simulink model "RobotLib"  (R2018b)
settings: Solver=ode5  StartTime=0.0  StopTime=10  FixedStep=0.0001  RelTol=1e-3
PreLoadFcn:
  | load('Arm6SimscapeData.mat');
model workspace: external: MAT-File E:\SixRobotArm\Simscape_Simulation\StepFile\Arm6Assembly_DataFile.mat (data not in the file)
values from neighbouring files (symbols this model uses):
  smiData =     [Arm6SimscapeData.mat]
undefined symbols (not defined in the file or in its folder): X, Y, Z
libraries: sm_lib x216, nesl_utility x186, fl_lib x114
(part 1 of 6)
settings Model: Creator=Administrator  LastModifiedBy=Jeason
settings SolverCC: AutoInsertRateTranBlk=on
settings DataIOCC: ReturnWorkspaceOutputs=on
settings ExplorerConfigSet: InternalSimMechanicsExplorerSettings="<ExplorerConfiguration><canonicalview>planar_xy</canonicalview><AnimationSetting><BasePlaybackSpeed>1.0</BasePlaybackSpeed><PlaybackSpeedFactor>1.0</PlaybackSpeedFactor></AnimationSetting><TilePanel><TileInfo><Tiles Columns=\"1\" Count=\"1\" Rows=\"1\"><Column Weight=\"1\"/><Row Weight=\"1\"/><Tile Height=\"1\" Width=\"1\" X=\"0\" Y=\"0\"/></Tiles></TileInfo><SceneInfo><SceneViewer><BGColor><R>0.60000002384185791</R><G>0.60000002384185791</G><B>0.60000002384185791</B></BGColor><Camera><DoPerspective>off</DoPerspective><Position><X>0.529425685588477024</X><Y>0.96968881474758839</Y><Z>0.531520526083879341</Z></Position><Center><X>-0.0479245836011489429</X><Y>0.392338545557962604</Y><Z>-0.0458297431057466537</Z></Center><Up><X>-0.408248290463863073</X><Y>0.816496580927726145</Y><Z>-0.408248290463863073</Z></Up><ViewLimDist>1</ViewLimDist><YLim>0.78131541566616991</YLim><XLim>0.557104420151891211</XLim></Camera></SceneViewer></SceneInfo></TilePanel><MechEditorPanel><Cameras/><GfxPanelCameraMap/><VideoCreator><PlaybackSpeedRatio>1.0</PlaybackSpeedRatio><FrameRate>30</FrameRate><VideoFormat>MPEG-4</VideoFormat><FrameSize>[400 400]</FrameSize></VideoCreator></MechEditorPanel></ExplorerConfiguration>"

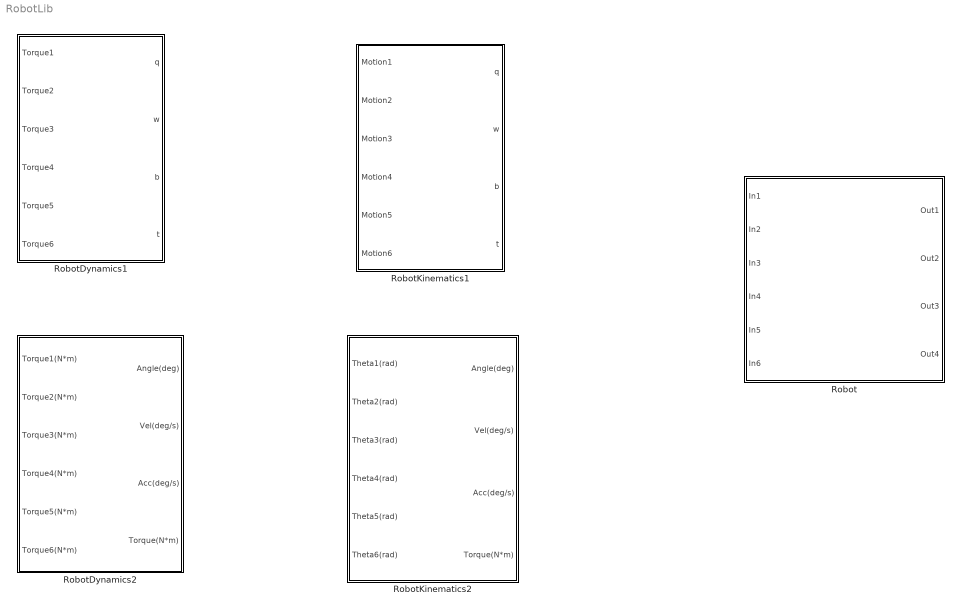
== system RobotLib ==
  Robot : Subsystem  mask(模式选择){VChoice=Kinematics}
      mask prompts: VChoice "Select a variant choice"
      mask help: 选择运动学Simscape模型或者动力学Simscape模型
      mask init:
      | %     simulationStatus =  get_param(bdroot,'SimulationStatus');
      | % 
      | % % The active variant can only be modified at edit-time or very early during
      | % % the simulink compile stage. 
      | %     choice = get_param(gcb,'VChoice');
      | %     vssBlk = [gcb, '/VariantSubsystem'];
      | %     oldVariant = get_param(gcb,'OverrideUsingVariant');
      | % 
      | %     if strcmp(choice,'Kinematics')
      | %         port_label('input', 1, 'Theta1(rad)');
      | %         port_label('input', 2, 'Theta2(rad)');
      | %         port_label('input', 3, 'Theta3(rad)');
      | %         port_label('input', 4, 'Theta4(rad)');
      | %         port_label('input', 5, 'Theta5(rad)');
      | %         port_label('input', 6, 'Theta6(rad)');
      | %         set_param(vssBlk, 'OverrideUsingVariant', 'Variant1');
      | %     else
      | %         port_label('input', 1, 'Torque1(N*m)');
      | %         port_label('input', 2, 'Torque2(N*m)');
      | %         port_label('input', 3, 'Torque3(N*m)');
      | %         port_label('input', 4, 'Torque4(N*m)');
      | %         port_label('input', 5, 'Torque5(N*m)');
      | %         port_label('input', 6, 'Torque6(N*m)');
      | %         set_param(vssBlk, 'OverrideUsingVariant', 'Variant2');
      | %     end
      mask TypeOptions VChoice: Kinematics | Dynamics
      mask Display:
      | image('E:\SixRobotArm\Robot.png') ;
      | simulationStatus =  get_param(bdroot,'SimulationStatus');
      | % The active variant can only be modified at edit-time or very early during
      | % the simulink compile stage.
      |     choice = get_param(gcb,'VChoice');
      |     vssBlk = [gcb, '/VariantSubsystem'];
      |     oldVariant = get_param(gcb,'OverrideUsingVariant');
      | if strcmp(choice,'Kinematics')
      |     port_label('input', 1, 'Theta1(rad)');
      |     port_label('input', 2, 'Theta2(rad)');
      |     port_label('input', 3, 'Theta3(rad)');
      |     port_label('input', 4, 'Theta4(rad)');
      |     port_label('input', 5, 'Theta5(rad)');
      |     port_label('input', 6, 'Theta6(rad)');
      |     set_param(vssBlk, 'OverrideUsingVariant', 'Variant1');
      | else
      |     port_label('input', 1, 'Torque1(N*m)');
      |     port_label('input', 2, 'Torque2(N*m)');
      |     port_label('input', 3, 'Torque3(N*m)');
      |     port_label('input', 4, 'Torque4(N*m)');
      |     port_label('input', 5, 'Torque5(N*m)');
      |     port_label('input', 6, 'Torque6(N*m)');
      |     set_param(vssBlk, 'OverrideUsingVariant', 'Variant2');
      | end
      | 
      | port_label('output', 1, 'Angle(deg)');
      | port_label('output', 2, 'Vel(deg/s)');
      | port_label('output', 3, 'Acc(deg/s^2)');
      | port_label('output', 4, 'Torque(N*m)');
  RobotDynamics1 : Subsystem
  RobotDynamics2 : Subsystem
  RobotKinematics1 : Subsystem
  RobotKinematics2 : Subsystem

== system RobotLib/Robot ==
  In1 : Inport
  In2 : Inport  Port=2
  In3 : Inport  Port=3
  In4 : Inport  Port=4
  In5 : Inport  Port=5
  In6 : Inport  Port=6
  VariantSubsystem : Subsystem  VariantControlMode=Label  Variant=on  LabelModeActiveChoice=Variant1
  Out1 : Outport
  Out2 : Outport  Port=2
  Out3 : Outport  Port=3
  Out4 : Outport  Port=4
  wires:
  VariantSubsystem/1(Out1) -> Out1/1
  In5/1 -> VariantSubsystem/5(In5)
  In1/1 -> VariantSubsystem/1(In1)
  In4/1 -> VariantSubsystem/4(In4)
  In6/1 -> VariantSubsystem/6(In6)
  In2/1 -> VariantSubsystem/2(In2)
  In3/1 -> VariantSubsystem/3(In3)
  VariantSubsystem/2(Out2) -> Out2/1
  VariantSubsystem/3(Out3) -> Out3/1
  VariantSubsystem/4(Out4) -> Out4/1

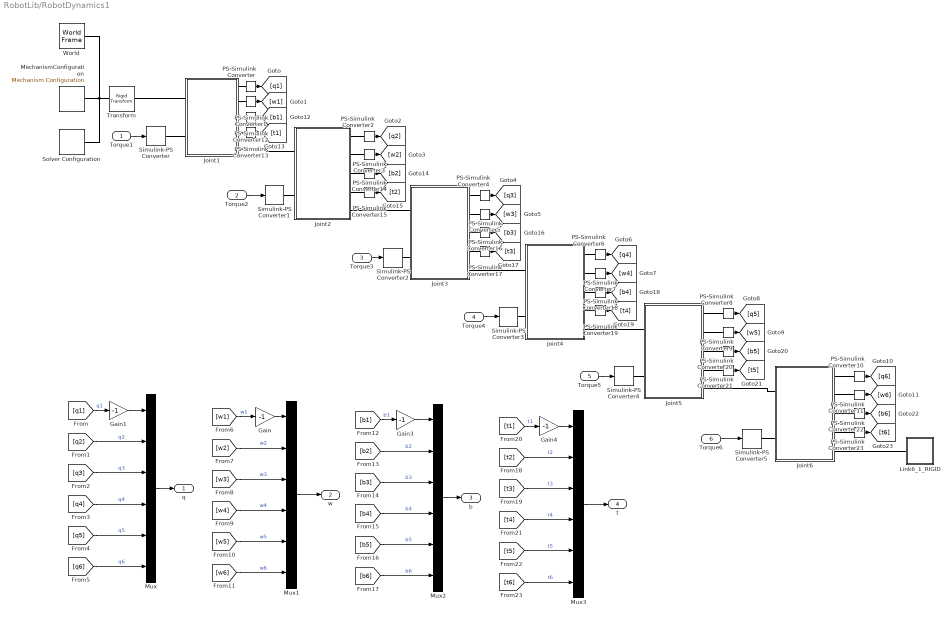
== system RobotLib/RobotDynamics1 ==
  Torque1 : Inport
  Torque2 : Inport  Port=2
  Torque3 : Inport  Port=3
  Torque4 : Inport  Port=4
  Torque5 : Inport  Port=5
  Torque6 : Inport  Port=6
  Gain{,1,3..4} (4 alike) : Gain  Gain=-1
  Joint1 : Subsystem
  Joint2 : Subsystem
  Joint3 : Subsystem
  Joint4 : Subsystem
  Joint5 : Subsystem
  Joint6 : Subsystem
  Link6_1_RIGID : Subsystem
  MechanismConfiguration : sm_lib/Utilities/Mechanism Configuration  UniformGravity=Constant  GravityVector=[0 -9.80665 0]  GravityUnits=m/s^2  LinearizationDelta=0.001
  Mux{,1..3} (4 alike) : Mux  Inputs=6
  PS-Simulink Converter{,2,4,6,8,10} (6 alike) : nesl_utility/PS-Simulink Converter  PhysicalDomain=network_engine_domain  SubClassName=ps_output  LeftPortType=input  RightPortType=output  PseudoPeriodic=off  Frequencies=[]  Unit=deg  AffineConversion=off
  PS-Simulink Converter{1,3,5,7,9,11} (6 alike) : nesl_utility/PS-Simulink Converter  PhysicalDomain=network_engine_domain  SubClassName=ps_output  LeftPortType=input  RightPortType=output  PseudoPeriodic=off  Frequencies=[]  Unit=deg/s  AffineConversion=off
  PS-Simulink Converter{12,14,16,18,20,22} (6 alike) : nesl_utility/PS-Simulink Converter  PhysicalDomain=network_engine_domain  SubClassName=ps_output  LeftPortType=input  RightPortType=output  PseudoPeriodic=off  Frequencies=[]  Unit=deg/s^2  AffineConversion=off
  PS-Simulink Converter{13,15,17,19,21,23} (6 alike) : nesl_utility/PS-Simulink Converter  PhysicalDomain=network_engine_domain  SubClassName=ps_output  LeftPortType=input  RightPortType=output  PseudoPeriodic=off  Frequencies=[]  Unit=N*m  AffineConversion=off
  Simulink-PS Converter{,1..5} (6 alike) : nesl_utility/Simulink-PS Converter  PhysicalDomain=network_engine_domain  SubClassName=ps_input  LeftPortType=input  RightPortType=output  PseudoPeriodic=off  Frequencies=[]  NoiseDistribution=none  NoiseParameters=[]  Unit=N*m  AffineConversion=off  FilteringAndDerivatives=provide  SimscapeFilterOrder=2  InputFilterTimeConstant=0.001  UdotUserProvided=0
  Solver Configuration : nesl_utility/Solver Configuration  PhysicalDomain=network_engine_domain  SubClassName=solver  LeftPortType=input  RightPortType=generic  Tones=[]  Harmonics=[]  SimulateNoise=off  Profile=off  UseLocalSampling=off  EnableSwitchedLinearOptims=on  FrequencyDomain=off  UseCCode=off  RelTol=0.001  AbsTol=1e-06  MinStep=1e-09  ToWorkspace=off  RevertToSquareIcSolve=off  NumHomotopyIterations=100  PhasorMode=off  PhasorModeNumHarmonics=1  DoDC=off  ResidualTolerance=1e-09  UseLocalSolver=off  LocalSolverChoice=NE_BACKWARD_EULER_ADVANCER  LocalSolverSampleTime=0.001  DoFixedCost=off  MaxNonlinIter=3  MaxModeIter=2  LinearAlgebra=auto  EquationFormulation=NE_TIME_EF  DelaysMemoryBudget=1024  AutomaticFiltering=on  FilteringTimeConstant=0.001  PartitionStorageMethod=AS_NEEDED  PartitionMemoryBudget=1024
  Transform : sm_lib/Frames and Transforms/Rigid Transform  TranslationMethod=Cartesian  TranslationStandardOffset=0  TranslationLengthUnit=mm  TranslationStandardAxis=+Z  TranslationCartesianOffset=smiData.RigidTransform(14).translation  TranslationROffset=0  TranslationROffsetUnits=m  TranslationZOffset=0  TranslationZOffsetUnits=m  TranslationThetaOffset=0  TranslationThetaOffsetUnits=deg  RotationMethod=ArbitraryAxis  RotationAngleUnits=rad  RotationStandardAxis=+Z  RotationAngle=smiData.RigidTransform(14).angle  RotationArbitraryAxis=smiData.RigidTransform(14).axis  FollAlignAxisA=+X  BaseAlignAxisA=+Y  FollAlignAxisB=+Y  BaseAlignAxisB=+Z  RotationSequenceAxes=FollowerAxes  RotationSequence=XYX  RotationSequenceAngles=[0 0 0]  RotationSequenceAnglesUnits=deg  RotationMatrix=[1 0 0; 0 1 0; 0 0 1]
  World : sm_lib/Frames and Transforms/World Frame
  q : Outport  VectorParamsAs1DForOutWhenUnconnected=on
  w : Outport  Port=2  VectorParamsAs1DForOutWhenUnconnected=on
  b : Outport  Port=3  VectorParamsAs1DForOutWhenUnconnected=on
  t : Outport  Port=4  VectorParamsAs1DForOutWhenUnconnected=on
  wires:
  [q5] -> Mux/5  "q5"
  Mux/1 -> q/1
  PS-Simulink Converter6/1 -> [q4]
  [w4] -> Mux1/4  "w4"
  PS-Simulink Converter/1 -> [q1]
  [q6] -> Mux/6  "q6"
  [w1] -> Gain/1  "w1"
  [w5] -> Mux1/5  "w5"
  PS-Simulink Converter4/1 -> [q3]
  PS-Simulink Converter5/1 -> [w3]
  PS-Simulink Converter9/1 -> [w5]
  [w2] -> Mux1/2  "w2"
  PS-Simulink Converter1/1 -> [w1]
  [q2] -> Mux/2  "q2"
  PS-Simulink Converter10/1 -> [q6]
  [w6] -> Mux1/6  "w6"
  PS-Simulink Converter7/1 -> [w4]
  [q4] -> Mux/4  "q4"
  PS-Simulink Converter11/1 -> [w6]
  PS-Simulink Converter8/1 -> [q5]
  Mux1/1 -> w/1
  PS-Simulink Converter2/1 -> [q2]
  [q3] -> Mux/3  "q3"
  [q1] -> Gain1/1  "q1"
  [w3] -> Mux1/3  "w3"
  PS-Simulink Converter3/1 -> [w2]
  Torque2/1 -> Simulink-PS Converter1/1
  Torque3/1 -> Simulink-PS Converter2/1
  Torque4/1 -> Simulink-PS Converter3/1
  Torque5/1 -> Simulink-PS Converter4/1
  Torque6/1 -> Simulink-PS Converter5/1
  Gain/1 -> Mux1/1
  Gain1/1 -> Mux/1
  PS-Simulink Converter12/1 -> [b1]
  PS-Simulink Converter13/1 -> [t1]
  PS-Simulink Converter15/1 -> [t2]
  PS-Simulink Converter14/1 -> [b2]
  PS-Simulink Converter16/1 -> [b3]
  PS-Simulink Converter17/1 -> [t3]
  PS-Simulink Converter19/1 -> [t4]
  PS-Simulink Converter18/1 -> [b4]
  PS-Simulink Converter20/1 -> [b5]
  PS-Simulink Converter21/1 -> [t5]
  PS-Simulink Converter23/1 -> [t6]
  PS-Simulink Converter22/1 -> [b6]
  Gain3/1 -> Mux2/1
  [b1] -> Gain3/1  "b1"
  Mux3/1 -> t/1
  [t1] -> Gain4/1  "t1"
  Mux2/1 -> b/1
  [b2] -> Mux2/2  "b2"
  [b3] -> Mux2/3  "b3"
  [b4] -> Mux2/4  "b4"
  [b5] -> Mux2/5  "b5"
  [b6] -> Mux2/6  "b6"
  [t2] -> Mux3/2  "t2"
  [t3] -> Mux3/3  "t3"
  [t4] -> Mux3/4  "t4"
  [t5] -> Mux3/5  "t5"
  [t6] -> Mux3/6  "t6"
  Torque1/1 -> Simulink-PS Converter/1
  Gain4/1 -> Mux3/1
  connections:
  Joint6/RConn1 -- PS-Simulink Converter10/LConn1
  PS-Simulink Converter11/LConn1 -- Joint6/RConn2
  Joint4/RConn2 -- PS-Simulink Converter7/LConn1
  Joint4/RConn1 -- PS-Simulink Converter6/LConn1
  PS-Simulink Converter9/LConn1 -- Joint5/RConn2
  PS-Simulink Converter5/LConn1 -- Joint3/RConn2
  Transform/LConn1 -- MechanismConfiguration/RConn1 -- Solver Configuration/RConn1 -- World/RConn1
  Joint3/RConn5 -- Joint4/LConn1
  Joint1/RConn2 -- PS-Simulink Converter1/LConn1
  PS-Simulink Converter3/LConn1 -- Joint2/RConn2
  Joint1/LConn1 -- Transform/RConn1
  PS-Simulink Converter8/LConn1 -- Joint5/RConn1
  Simulink-PS Converter3/RConn1 -- Joint4/LConn2
  PS-Simulink Converter4/LConn1 -- Joint3/RConn1
  Joint1/RConn1 -- PS-Simulink Converter/LConn1
  Joint6/LConn1 -- Joint5/RConn5
  Joint3/LConn1 -- Joint2/RConn5
  Joint5/LConn1 -- Joint4/RConn5
  Link6_1_RIGID/LConn1 -- Joint6/RConn5
  Simulink-PS Converter5/RConn1 -- Joint6/LConn2
  Simulink-PS Converter1/RConn1 -- Joint2/LConn2
  PS-Simulink Converter2/LConn1 -- Joint2/RConn1
  Joint5/LConn2 -- Simulink-PS Converter4/RConn1
  Joint2/LConn1 -- Joint1/RConn5
  Simulink-PS Converter2/RConn1 -- Joint3/LConn2
  PS-Simulink Converter12/LConn1 -- Joint1/RConn3
  PS-Simulink Converter13/LConn1 -- Joint1/RConn4
  PS-Simulink Converter15/LConn1 -- Joint2/RConn4
  PS-Simulink Converter14/LConn1 -- Joint2/RConn3
  PS-Simulink Converter16/LConn1 -- Joint3/RConn3
  Joint3/RConn4 -- PS-Simulink Converter17/LConn1
  PS-Simulink Converter18/LConn1 -- Joint4/RConn3
  PS-Simulink Converter19/LConn1 -- Joint4/RConn4
  PS-Simulink Converter20/LConn1 -- Joint5/RConn3
  PS-Simulink Converter21/LConn1 -- Joint5/RConn4
  PS-Simulink Converter23/LConn1 -- Joint6/RConn4
  Joint6/RConn3 -- PS-Simulink Converter22/LConn1
  Joint1/LConn2 -- Simulink-PS Converter/RConn1

== system RobotLib/RobotDynamics2 ==
  Torque1(N*m) : Inport
  Torque2(N*m) : Inport  Port=2
  Torque3(N*m) : Inport  Port=3
  Torque4(N*m) : Inport  Port=4
  Torque5(N*m) : Inport  Port=5
  Torque6(N*m) : Inport  Port=6
  RobotDynamics1 : Subsystem
  Angle(deg) : Outport
  Vel(deg/s) : Outport  Port=2
  Acc(deg/s) : Outport  Port=3
  Torque(N*m) : Outport  Port=4
  wires:
  Torque5(N*m)/1 -> RobotDynamics1/5(Torque5)
  Torque2(N*m)/1 -> RobotDynamics1/2(Torque2)
  Torque3(N*m)/1 -> RobotDynamics1/3(Torque3)
  Torque6(N*m)/1 -> RobotDynamics1/6(Torque6)
  RobotDynamics1/1(q) -> Angle(deg)/1
  Torque1(N*m)/1 -> RobotDynamics1/1(Torque1)
  Torque4(N*m)/1 -> RobotDynamics1/4(Torque4)
  RobotDynamics1/2(w) -> Vel(deg/s)/1
  RobotDynamics1/3(b) -> Acc(deg/s)/1
  RobotDynamics1/4(t) -> Torque(N*m)/1

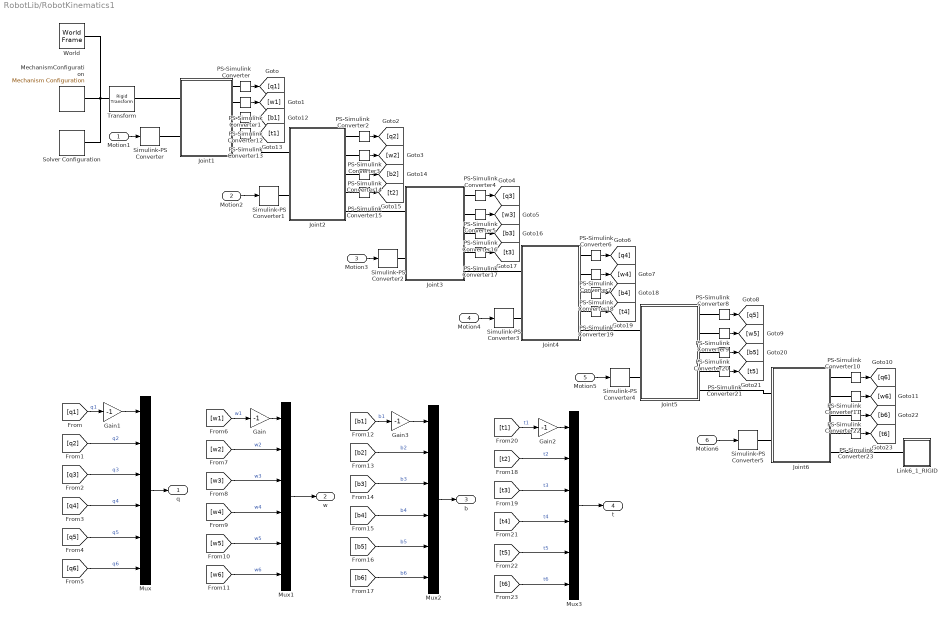
== system RobotLib/RobotKinematics1 ==
  Motion1 : Inport
  Motion2 : Inport  Port=2
  Motion3 : Inport  Port=3
  Motion4 : Inport  Port=4
  Motion5 : Inport  Port=5
  Motion6 : Inport  Port=6
  Gain{,1..3} (4 alike) : Gain  Gain=-1
  Joint1 : Subsystem
  Joint2 : Subsystem
  Joint3 : Subsystem
  Joint4 : Subsystem
  Joint5 : Subsystem
  Joint6 : Subsystem
  Link6_1_RIGID : Subsystem
  MechanismConfiguration : sm_lib/Utilities/Mechanism Configuration  UniformGravity=Constant  GravityVector=[0 -9.80665 0]  GravityUnits=m/s^2  LinearizationDelta=0.001
  Mux{,1..3} (4 alike) : Mux  Inputs=6
  PS-Simulink Converter{,2,4,6,8,10} (6 alike) : nesl_utility/PS-Simulink Converter  PhysicalDomain=network_engine_domain  SubClassName=ps_output  LeftPortType=input  RightPortType=output  PseudoPeriodic=off  Frequencies=[]  Unit=deg  AffineConversion=off
  PS-Simulink Converter{1,3,5,7,9,11} (6 alike) : nesl_utility/PS-Simulink Converter  PhysicalDomain=network_engine_domain  SubClassName=ps_output  LeftPortType=input  RightPortType=output  PseudoPeriodic=off  Frequencies=[]  Unit=deg/s  AffineConversion=off
  PS-Simulink Converter{12,14,16,18,20,22} (6 alike) : nesl_utility/PS-Simulink Converter  PhysicalDomain=network_engine_domain  SubClassName=ps_output  LeftPortType=input  RightPortType=output  PseudoPeriodic=off  Frequencies=[]  Unit=deg/s^2  AffineConversion=off
  PS-Simulink Converter{13,15,17,19,21,23} (6 alike) : nesl_utility/PS-Simulink Converter  PhysicalDomain=network_engine_domain  SubClassName=ps_output  LeftPortType=input  RightPortType=output  PseudoPeriodic=off  Frequencies=[]  Unit=N*m  AffineConversion=off
  Simulink-PS Converter{,1..5} (6 alike) : nesl_utility/Simulink-PS Converter  PhysicalDomain=network_engine_domain  SubClassName=ps_input  LeftPortType=input  RightPortType=output  PseudoPeriodic=off  Frequencies=[]  NoiseDistribution=none  NoiseParameters=[]  Unit=rad  AffineConversion=off  FilteringAndDerivatives=provide  SimscapeFilterOrder=2  InputFilterTimeConstant=0.001  UdotUserProvided=0
  Solver Configuration : nesl_utility/Solver Configuration  PhysicalDomain=network_engine_domain  SubClassName=solver  LeftPortType=input  RightPortType=generic  Tones=[]  Harmonics=[]  SimulateNoise=off  Profile=off  UseLocalSampling=off  EnableSwitchedLinearOptims=on  FrequencyDomain=off  UseCCode=off  RelTol=0.001  AbsTol=1e-06  MinStep=1e-09  ToWorkspace=off  RevertToSquareIcSolve=off  NumHomotopyIterations=100  PhasorMode=off  PhasorModeNumHarmonics=1  DoDC=off  ResidualTolerance=1e-09  UseLocalSolver=off  LocalSolverChoice=NE_BACKWARD_EULER_ADVANCER  LocalSolverSampleTime=0.001  DoFixedCost=off  MaxNonlinIter=3  MaxModeIter=2  LinearAlgebra=auto  EquationFormulation=NE_TIME_EF  DelaysMemoryBudget=1024  AutomaticFiltering=on  FilteringTimeConstant=0.001  PartitionStorageMethod=AS_NEEDED  PartitionMemoryBudget=1024
  Transform : sm_lib/Frames and Transforms/Rigid Transform  TranslationMethod=Cartesian  TranslationStandardOffset=0  TranslationLengthUnit=mm  TranslationStandardAxis=+Z  TranslationCartesianOffset=smiData.RigidTransform(14).translation  TranslationROffset=0  TranslationROffsetUnits=m  TranslationZOffset=0  TranslationZOffsetUnits=m  TranslationThetaOffset=0  TranslationThetaOffsetUnits=deg  RotationMethod=ArbitraryAxis  RotationAngleUnits=rad  RotationStandardAxis=+Z  RotationAngle=smiData.RigidTransform(14).angle  RotationArbitraryAxis=smiData.RigidTransform(14).axis  FollAlignAxisA=+X  BaseAlignAxisA=+Y  FollAlignAxisB=+Y  BaseAlignAxisB=+Z  RotationSequenceAxes=FollowerAxes  RotationSequence=XYX  RotationSequenceAngles=[0 0 0]  RotationSequenceAnglesUnits=deg  RotationMatrix=[1 0 0; 0 1 0; 0 0 1]
  World : sm_lib/Frames and Transforms/World Frame
  q : Outport  VectorParamsAs1DForOutWhenUnconnected=on
  w : Outport  Port=2  VectorParamsAs1DForOutWhenUnconnected=on
  b : Outport  Port=3  VectorParamsAs1DForOutWhenUnconnected=on
  t : Outport  Port=4  VectorParamsAs1DForOutWhenUnconnected=on
  wires:
  [t6] -> Mux3/6  "t6"
  [t5] -> Mux3/5  "t5"
  [t4] -> Mux3/4  "t4"
  [t3] -> Mux3/3  "t3"
  [t2] -> Mux3/2  "t2"
  [b6] -> Mux2/6  "b6"
  [b5] -> Mux2/5  "b5"
  [b4] -> Mux2/4  "b4"
  [b3] -> Mux2/3  "b3"
  [b2] -> Mux2/2  "b2"
  Mux2/1 -> b/1
  [t1] -> Gain2/1  "t1"
  Mux3/1 -> t/1
  [b1] -> Gain3/1  "b1"
  Gain2/1 -> Mux3/1
  Gain3/1 -> Mux2/1
  PS-Simulink Converter22/1 -> [b6]
  PS-Simulink Converter23/1 -> [t6]
  PS-Simulink Converter21/1 -> [t5]
  PS-Simulink Converter20/1 -> [b5]
  PS-Simulink Converter18/1 -> [b4]
  PS-Simulink Converter19/1 -> [t4]
  PS-Simulink Converter17/1 -> [t3]
  PS-Simulink Converter16/1 -> [b3]
  PS-Simulink Converter14/1 -> [b2]
  PS-Simulink Converter15/1 -> [t2]
  PS-Simulink Converter13/1 -> [t1]
  PS-Simulink Converter12/1 -> [b1]
  Gain1/1 -> Mux/1
  Gain/1 -> Mux1/1
  Motion6/1 -> Simulink-PS Converter5/1
  Motion5/1 -> Simulink-PS Converter4/1
  Motion4/1 -> Simulink-PS Converter3/1
  Motion3/1 -> Simulink-PS Converter2/1
  Motion2/1 -> Simulink-PS Converter1/1
  Motion1/1 -> Simulink-PS Converter/1
  PS-Simulink Converter3/1 -> [w2]
  [w3] -> Mux1/3  "w3"
  [q1] -> Gain1/1  "q1"
  [q3] -> Mux/3  "q3"
  PS-Simulink Converter2/1 -> [q2]
  Mux1/1 -> w/1
  PS-Simulink Converter8/1 -> [q5]
  PS-Simulink Converter11/1 -> [w6]
  [q4] -> Mux/4  "q4"
  PS-Simulink Converter7/1 -> [w4]
  [w6] -> Mux1/6  "w6"
  PS-Simulink Converter10/1 -> [q6]
  [q2] -> Mux/2  "q2"
  PS-Simulink Converter1/1 -> [w1]
  [w2] -> Mux1/2  "w2"
  PS-Simulink Converter9/1 -> [w5]
  PS-Simulink Converter5/1 -> [w3]
  PS-Simulink Converter4/1 -> [q3]
  [w5] -> Mux1/5  "w5"
  [w1] -> Gain/1  "w1"
  [q6] -> Mux/6  "q6"
  PS-Simulink Converter/1 -> [q1]
  [w4] -> Mux1/4  "w4"
  PS-Simulink Converter6/1 -> [q4]
  Mux/1 -> q/1
  [q5] -> Mux/5  "q5"
  connections:
  Joint6/RConn3 -- PS-Simulink Converter22/LConn1
  PS-Simulink Converter23/LConn1 -- Joint6/RConn4
  PS-Simulink Converter21/LConn1 -- Joint5/RConn4
  PS-Simulink Converter20/LConn1 -- Joint5/RConn3
  PS-Simulink Converter19/LConn1 -- Joint4/RConn4
  PS-Simulink Converter18/LConn1 -- Joint4/RConn3
  Joint3/RConn4 -- PS-Simulink Converter17/LConn1
  PS-Simulink Converter16/LConn1 -- Joint3/RConn3
  PS-Simulink Converter14/LConn1 -- Joint2/RConn3
  PS-Simulink Converter15/LConn1 -- Joint2/RConn4
  PS-Simulink Converter13/LConn1 -- Joint1/RConn4
  PS-Simulink Converter12/LConn1 -- Joint1/RConn3
  Joint1/LConn2 -- Simulink-PS Converter/RConn1
  Simulink-PS Converter2/RConn1 -- Joint3/LConn2
  Joint2/LConn1 -- Joint1/RConn5
  Joint5/LConn2 -- Simulink-PS Converter4/RConn1
  PS-Simulink Converter2/LConn1 -- Joint2/RConn1
  Simulink-PS Converter1/RConn1 -- Joint2/LConn2
  Simulink-PS Converter5/RConn1 -- Joint6/LConn2
  Link6_1_RIGID/LConn1 -- Joint6/RConn5
  Joint5/LConn1 -- Joint4/RConn5
  Joint3/LConn1 -- Joint2/RConn5
  Joint6/LConn1 -- Joint5/RConn5
  Joint1/RConn1 -- PS-Simulink Converter/LConn1
  PS-Simulink Converter4/LConn1 -- Joint3/RConn1
  Simulink-PS Converter3/RConn1 -- Joint4/LConn2
  PS-Simulink Converter8/LConn1 -- Joint5/RConn1
  Joint1/LConn1 -- Transform/RConn1
  PS-Simulink Converter3/LConn1 -- Joint2/RConn2
  Joint1/RConn2 -- PS-Simulink Converter1/LConn1
  Joint3/RConn5 -- Joint4/LConn1
  World/RConn1 -- Solver Configuration/RConn1 -- MechanismConfiguration/RConn1 -- Transform/LConn1
  PS-Simulink Converter5/LConn1 -- Joint3/RConn2
  PS-Simulink Converter9/LConn1 -- Joint5/RConn2
  Joint4/RConn1 -- PS-Simulink Converter6/LConn1
  Joint4/RConn2 -- PS-Simulink Converter7/LConn1
  PS-Simulink Converter11/LConn1 -- Joint6/RConn2
  Joint6/RConn1 -- PS-Simulink Converter10/LConn1

== system RobotLib/RobotKinematics2 ==
  Theta1(rad) : Inport
  Theta2(rad) : Inport  Port=2
  Theta3(rad) : Inport  Port=3
  Theta4(rad) : Inport  Port=4
  Theta5(rad) : Inport  Port=5
  Theta6(rad) : Inport  Port=6
  RobotKinematics1 : Subsystem
  Angle(deg) : Outport
  Vel(deg/s) : Outport  Port=2
  Acc(deg/s) : Outport  Port=3
  Torque(N*m) : Outport  Port=4
  wires:
  Theta4(rad)/1 -> RobotKinematics1/4(Motion4)
  RobotKinematics1/1(q) -> Angle(deg)/1
  Theta1(rad)/1 -> RobotKinematics1/1(Motion1)
  Theta2(rad)/1 -> RobotKinematics1/2(Motion2)
  Theta3(rad)/1 -> RobotKinematics1/3(Motion3)
  Theta5(rad)/1 -> RobotKinematics1/5(Motion5)
  RobotKinematics1/3(b) -> Acc(deg/s)/1
  RobotKinematics1/2(w) -> Vel(deg/s)/1
  Theta6(rad)/1 -> RobotKinematics1/6(Motion6)
  RobotKinematics1/4(t) -> Torque(N*m)/1

== system RobotLib/Robot/VariantSubsystem ==
  note: 1) Add Subsystem or Model blocks as valid variant choices.
      | 2) You cannot connect blocks at this level. At simulation, connectivity is automatically
      | determined, based on the active variant and port name matching.
  In1 : Inport
  In2 : Inport  Port=2
  In3 : Inport  Port=3
  In4 : Inport  Port=4
  In5 : Inport  Port=5
  In6 : Inport  Port=6
  Subsystem : Subsystem  VariantControl=Variant2
  Subsystem1 : Subsystem  VariantControl=Variant1
  Out1 : Outport
  Out2 : Outport  Port=2
  Out3 : Outport  Port=3
  Out4 : Outport  Port=4

== system RobotLib/RobotDynamics1/Joint1 ==
  note: 初始角度
  BaseBracket_1_RIGID : Subsystem
  PS Constant1 : fl_lib/Physical Signals/Sources/PS Constant  constant=-pi/2
  PS Gain : fl_lib/Physical Signals/Functions/PS Gain  gain=-1
  PS Subtract1 : fl_lib/Physical Signals/Functions/PS Subtract
      settings: SourceProductName=Simscape
  Revolute1 : sm_lib/Joints/Revolute Joint  SenseConstraintForce=off  SenseConstraintForceX=off  SenseConstraintForceY=off  SenseConstraintForceZ=off  SenseConstraintTorque=off  SenseConstraintTorqueX=off  SenseConstraintTorqueY=off  SenseConstraintTorqueZ=off  SenseTotalForce=off  SenseTotalForceX=off  SenseTotalForceY=off  SenseTotalForceZ=off  SenseTotalTorque=off  SenseTotalTorqueX=off  SenseTotalTorqueY=off  SenseTotalTorqueZ=off  CompositeWrenchDir=FollowerOnBase  CompositeWrenchFrame=BaseFrame  EquilibriumPosition=0  EquilibriumPositionUnits=rad  SpringStiffness=0  SpringStiffnessUnits=N*m/rad  DampingCoefficient=0  DampingCoefficientUnits=N*m/(rad/s)  TorqueActuationMode=InputTorque  MotionActuationMode=ComputedMotion  SensePosition=on  SenseVelocity=on  SenseAcceleration=on  SenseTorqueForce=on  PositionTargetSpecify=on  PositionTargetPriority=Low  PositionTargetValue=smiData.RevoluteJoint(2).Rz.Pos  PositionTargetValueUnits=deg  VelocityTargetSpecify=off  VelocityTargetPriority=High  VelocityTargetValue=0  VelocityTargetValueUnits=deg/s
  BaseConn : PMIOPort  Side=Left
  Torque1 : PMIOPort  Port=2  Side=Left
  q1 : PMIOPort  Port=3  Side=Right
  w1 : PMIOPort  Port=4  Side=Right
  b1 : PMIOPort  Port=5  Side=Right
  t1 : PMIOPort  Port=6  Side=Right
  Conn1 : PMIOPort  Port=7  Side=Right
  connections:
  BaseBracket_1_RIGID/RConn1 -- Revolute1/LConn1
  Conn1/RConn1 -- Revolute1/RConn1
  BaseBracket_1_RIGID/LConn1 -- BaseConn/RConn1
  PS Subtract1/LConn1 -- Revolute1/RConn2
  PS Constant1/RConn1 -- PS Subtract1/LConn2
  PS Subtract1/RConn1 -- q1/RConn1
  Revolute1/RConn3 -- w1/RConn1
  Torque1/RConn1 -- PS Gain/LConn1
  b1/RConn1 -- Revolute1/RConn4
  t1/RConn1 -- Revolute1/RConn5
  PS Gain/RConn1 -- Revolute1/LConn2

== system RobotLib/RobotDynamics1/Joint2 ==
  note: 初始角度
  Link1_2_RIGID : Subsystem
  PS Constant2 : fl_lib/Physical Signals/Sources/PS Constant  constant=-pi/2
  PS Subtract1 : fl_lib/Physical Signals/Functions/PS Subtract
      settings: SourceProductName=Simscape
  Revolute : sm_lib/Joints/Revolute Joint  SenseConstraintForce=off  SenseConstraintForceX=off  SenseConstraintForceY=off  SenseConstraintForceZ=off  SenseConstraintTorque=off  SenseConstraintTorqueX=off  SenseConstraintTorqueY=off  SenseConstraintTorqueZ=off  SenseTotalForce=off  SenseTotalForceX=off  SenseTotalForceY=off  SenseTotalForceZ=off  SenseTotalTorque=off  SenseTotalTorqueX=off  SenseTotalTorqueY=off  SenseTotalTorqueZ=off  CompositeWrenchDir=FollowerOnBase  CompositeWrenchFrame=BaseFrame  EquilibriumPosition=0  EquilibriumPositionUnits=rad  SpringStiffness=0  SpringStiffnessUnits=N*m/rad  DampingCoefficient=0  DampingCoefficientUnits=N*m/(rad/s)  TorqueActuationMode=InputTorque  MotionActuationMode=ComputedMotion  SensePosition=on  SenseVelocity=on  SenseAcceleration=on  SenseTorqueForce=on  PositionTargetSpecify=on  PositionTargetPriority=Low  PositionTargetValue=smiData.RevoluteJoint(1).Rz.Pos  PositionTargetValueUnits=deg  VelocityTargetSpecify=off  VelocityTargetPriority=High  VelocityTargetValue=0  VelocityTargetValueUnits=deg/s
  Conn1 : PMIOPort  Side=Left
  q2 : PMIOPort  Port=2  Side=Right
  Torque2 : PMIOPort  Port=3  Side=Left
  w2 : PMIOPort  Port=4  Side=Right
  b2 : PMIOPort  Port=5  Side=Right
  t2 : PMIOPort  Port=6  Side=Right
  Conn2 : PMIOPort  Port=7  Side=Right
  connections:
  Link1_2_RIGID/LConn1 -- Conn1/RConn1
  Link1_2_RIGID/RConn1 -- Revolute/LConn1
  Conn2/RConn1 -- Revolute/RConn1
  PS Subtract1/LConn1 -- Revolute/RConn2
  Revolute/RConn3 -- w2/RConn1
  Torque2/RConn1 -- Revolute/LConn2
  PS Constant2/RConn1 -- PS Subtract1/LConn2
  PS Subtract1/RConn1 -- q2/RConn1
  b2/RConn1 -- Revolute/RConn4
  t2/RConn1 -- Revolute/RConn5

== system RobotLib/RobotDynamics1/Joint3 ==
  note: 初始角度
  Link2_2_RIGID : Subsystem
  PS Constant2 : fl_lib/Physical Signals/Sources/PS Constant  constant=0
  PS Subtract1 : fl_lib/Physical Signals/Functions/PS Subtract
      settings: SourceProductName=Simscape
  Revolute2 : sm_lib/Joints/Revolute Joint  SenseConstraintForce=off  SenseConstraintForceX=off  SenseConstraintForceY=off  SenseConstraintForceZ=off  SenseConstraintTorque=off  SenseConstraintTorqueX=off  SenseConstraintTorqueY=off  SenseConstraintTorqueZ=off  SenseTotalForce=off  SenseTotalForceX=off  SenseTotalForceY=off  SenseTotalForceZ=off  SenseTotalTorque=off  SenseTotalTorqueX=off  SenseTotalTorqueY=off  SenseTotalTorqueZ=off  CompositeWrenchDir=FollowerOnBase  CompositeWrenchFrame=BaseFrame  EquilibriumPosition=0  EquilibriumPositionUnits=rad  SpringStiffness=0  SpringStiffnessUnits=N*m/rad  DampingCoefficient=0  DampingCoefficientUnits=N*m/(rad/s)  TorqueActuationMode=InputTorque  MotionActuationMode=ComputedMotion  SensePosition=on  SenseVelocity=on  SenseAcceleration=on  SenseTorqueForce=on  PositionTargetSpecify=on  PositionTargetPriority=Low  PositionTargetValue=smiData.RevoluteJoint(3).Rz.Pos  PositionTargetValueUnits=deg  VelocityTargetSpecify=off  VelocityTargetPriority=High  VelocityTargetValue=0  VelocityTargetValueUnits=deg/s
  Conn2 : PMIOPort  Side=Left
  Torque3 : PMIOPort  Port=2  Side=Left
  q3 : PMIOPort  Port=3  Side=Right
  w3 : PMIOPort  Port=4  Side=Right
  w1 : PMIOPort  Port=5  Side=Right
  w2 : PMIOPort  Port=6  Side=Right
  Conn3 : PMIOPort  Port=7  Side=Right
  connections:
  Link2_2_RIGID/RConn1 -- Revolute2/LConn1
  Link2_2_RIGID/LConn1 -- Conn2/RConn1
  Revolute2/LConn2 -- Torque3/RConn1
  Conn3/RConn1 -- Revolute2/RConn1
  PS Subtract1/LConn2 -- PS Constant2/RConn1
  PS Subtract1/RConn1 -- q3/RConn1
  PS Subtract1/LConn1 -- Revolute2/RConn2
  w3/RConn1 -- Revolute2/RConn3
  w1/RConn1 -- Revolute2/RConn4
  w2/RConn1 -- Revolute2/RConn5

== system RobotLib/RobotDynamics1/Joint4 ==
  note: 初始角度
  Link3_1_RIGID : Subsystem
  PS Constant2 : fl_lib/Physical Signals/Sources/PS Constant  constant=0
  PS Subtract1 : fl_lib/Physical Signals/Functions/PS Subtract
      settings: SourceProductName=Simscape
  Revolute3 : sm_lib/Joints/Revolute Joint  SenseConstraintForce=off  SenseConstraintForceX=off  SenseConstraintForceY=off  SenseConstraintForceZ=off  SenseConstraintTorque=off  SenseConstraintTorqueX=off  SenseConstraintTorqueY=off  SenseConstraintTorqueZ=off  SenseTotalForce=off  SenseTotalForceX=off  SenseTotalForceY=off  SenseTotalForceZ=off  SenseTotalTorque=off  SenseTotalTorqueX=off  SenseTotalTorqueY=off  SenseTotalTorqueZ=off  CompositeWrenchDir=FollowerOnBase  CompositeWrenchFrame=BaseFrame  EquilibriumPosition=0  EquilibriumPositionUnits=rad  SpringStiffness=0  SpringStiffnessUnits=N*m/rad  DampingCoefficient=0  DampingCoefficientUnits=N*m/(rad/s)  TorqueActuationMode=InputTorque  MotionActuationMode=ComputedMotion  SensePosition=on  SenseVelocity=on  SenseAcceleration=on  SenseTorqueForce=on  PositionTargetSpecify=on  PositionTargetPriority=Low  PositionTargetValue=smiData.RevoluteJoint(4).Rz.Pos  PositionTargetValueUnits=deg  VelocityTargetSpecify=off  VelocityTargetPriority=High  VelocityTargetValue=0  VelocityTargetValueUnits=deg/s
  Conn3 : PMIOPort  Side=Left
  Torque4 : PMIOPort  Port=2  Side=Left
  q4 : PMIOPort  Port=3  Side=Right
  w4 : PMIOPort  Port=4  Side=Right
  b4 : PMIOPort  Port=5  Side=Right
  t4 : PMIOPort  Port=6  Side=Right
  Conn4 : PMIOPort  Port=7  Side=Right
  connections:
  Torque4/RConn1 -- Revolute3/LConn2
  Link3_1_RIGID/RConn1 -- Revolute3/LConn1
  Link3_1_RIGID/LConn1 -- Conn3/RConn1
  PS Subtract1/LConn1 -- Revolute3/RConn2
  PS Subtract1/RConn1 -- q4/RConn1
  PS Constant2/RConn1 -- PS Subtract1/LConn2
  Conn4/RConn1 -- Revolute3/RConn1
  w4/RConn1 -- Revolute3/RConn3
  b4/RConn1 -- Revolute3/RConn4
  t4/RConn1 -- Revolute3/RConn5

== system RobotLib/RobotDynamics1/Joint5 ==
  note: 初始角度
  Link4_1_RIGID : Subsystem
  PS Constant2 : fl_lib/Physical Signals/Sources/PS Constant  constant=pi/2
  PS Subtract1 : fl_lib/Physical Signals/Functions/PS Subtract
      settings: SourceProductName=Simscape
  Revolute5 : sm_lib/Joints/Revolute Joint  SenseConstraintForce=off  SenseConstraintForceX=off  SenseConstraintForceY=off  SenseConstraintForceZ=off  SenseConstraintTorque=off  SenseConstraintTorqueX=off  SenseConstraintTorqueY=off  SenseConstraintTorqueZ=off  SenseTotalForce=off  SenseTotalForceX=off  SenseTotalForceY=off  SenseTotalForceZ=off  SenseTotalTorque=off  SenseTotalTorqueX=off  SenseTotalTorqueY=off  SenseTotalTorqueZ=off  CompositeWrenchDir=FollowerOnBase  CompositeWrenchFrame=BaseFrame  EquilibriumPosition=0  EquilibriumPositionUnits=rad  SpringStiffness=0  SpringStiffnessUnits=N*m/rad  DampingCoefficient=0  DampingCoefficientUnits=N*m/(rad/s)  TorqueActuationMode=InputTorque  MotionActuationMode=ComputedMotion  SensePosition=on  SenseVelocity=on  SenseAcceleration=on  SenseTorqueForce=on  PositionTargetSpecify=on  PositionTargetPriority=Low  PositionTargetValue=smiData.RevoluteJoint(5).Rz.Pos  PositionTargetValueUnits=deg  VelocityTargetSpecify=off  VelocityTargetPriority=High  VelocityTargetValue=0  VelocityTargetValueUnits=deg/s
  Conn4 : PMIOPort  Side=Left
  Torque : PMIOPort  Port=2  Side=Left
  q5 : PMIOPort  Port=3  Side=Right
  w5 : PMIOPort  Port=4  Side=Right
  b5 : PMIOPort  Port=5  Side=Right
  t5 : PMIOPort  Port=6  Side=Right
  Conn5 : PMIOPort  Port=7  Side=Right
  connections:
  Link4_1_RIGID/RConn1 -- Revolute5/LConn1
  Revolute5/LConn2 -- Torque/RConn1
  Link4_1_RIGID/LConn1 -- Conn4/RConn1
  PS Subtract1/LConn1 -- Revolute5/RConn2
  PS Subtract1/RConn1 -- q5/RConn1
  PS Subtract1/LConn2 -- PS Constant2/RConn1
  Conn5/RConn1 -- Revolute5/RConn1
  w5/RConn1 -- Revolute5/RConn3
  b5/RConn1 -- Revolute5/RConn4
  t5/RConn1 -- Revolute5/RConn5

== system RobotLib/RobotDynamics1/Joint6 ==
  note: 初始角度
  Link5_2_RIGID : Subsystem
  PS Constant2 : fl_lib/Physical Signals/Sources/PS Constant  constant=-pi
  PS Subtract1 : fl_lib/Physical Signals/Functions/PS Subtract
      settings: SourceProductName=Simscape
  Revolute6 : sm_lib/Joints/Revolute Joint  SenseConstraintForce=off  SenseConstraintForceX=off  SenseConstraintForceY=off  SenseConstraintForceZ=off  SenseConstraintTorque=off  SenseConstraintTorqueX=off  SenseConstraintTorqueY=off  SenseConstraintTorqueZ=off  SenseTotalForce=off  SenseTotalForceX=off  SenseTotalForceY=off  SenseTotalForceZ=off  SenseTotalTorque=off  SenseTotalTorqueX=off  SenseTotalTorqueY=off  SenseTotalTorqueZ=off  CompositeWrenchDir=FollowerOnBase  CompositeWrenchFrame=BaseFrame  EquilibriumPosition=0  EquilibriumPositionUnits=rad  SpringStiffness=0  SpringStiffnessUnits=N*m/rad  DampingCoefficient=0  DampingCoefficientUnits=N*m/(rad/s)  TorqueActuationMode=InputTorque  MotionActuationMode=ComputedMotion  SensePosition=on  SenseVelocity=on  SenseAcceleration=on  SenseTorqueForce=on  PositionTargetSpecify=on  PositionTargetPriority=Low  PositionTargetValue=smiData.RevoluteJoint(6).Rz.Pos  PositionTargetValueUnits=deg  VelocityTargetSpecify=off  VelocityTargetPriority=High  VelocityTargetValue=0  VelocityTargetValueUnits=deg/s
  Conn5 : PMIOPort  Side=Left
  Torque6 : PMIOPort  Port=2  Side=Left
  q6 : PMIOPort  Port=3  Side=Right
  w6 : PMIOPort  Port=4  Side=Right
  b6 : PMIOPort  Port=5  Side=Right
  t6 : PMIOPort  Port=6  Side=Right
  Conn6 : PMIOPort  Port=7  Side=Right
  connections:
  Link5_2_RIGID/RConn1 -- Revolute6/LConn1
  Link5_2_RIGID/LConn1 -- Conn5/RConn1
  PS Subtract1/LConn1 -- Revolute6/RConn2
  Revolute6/LConn2 -- Torque6/RConn1
  PS Subtract1/RConn1 -- q6/RConn1
  PS Subtract1/LConn2 -- PS Constant2/RConn1
  Conn6/RConn1 -- Revolute6/RConn1
  w6/RConn1 -- Revolute6/RConn3
  b6/RConn1 -- Revolute6/RConn4
  t6/RConn1 -- Revolute6/RConn5

== system RobotLib/RobotDynamics1/Link6_1_RIGID ==
  ReferenceFrame : sm_lib/Frames and Transforms/Reference Frame
  Solid : sm_lib/Body Elements/Solid  InertiaType=Custom  Mass=smiData.Solid(6).mass  MassUnits=kg  CenterOfMass=smiData.Solid(6).CoM  CenterOfMassUnits=mm  MomentsOfInertia=smiData.Solid(6).MoI  MomentsOfInertiaUnits=kg*mm^2  ProductsOfInertia=smiData.Solid(6).PoI  ProductsOfInertiaUnits=kg*mm^2  BasedOnType=DensityFromFile  Density=1000  DensityUnits=kg/m^3  DoExposeReferenceFrame=on  SerializedFrames=<Frames/>  GraphicType=FromGeometry  MarkerShape=Sphere  MarkerSize=10  GraphicVisPropType=SimpleVisualProperties  GraphicDiffuseColor=smiData.Solid(6).color  GraphicSpecularColor=[0.5 0.5 0.5 1.0]  GraphicAmbientColor=[0.15 0.15 0.15 1.0]  GraphicEmissiveColor=[0.0 0.0 0.0 1.0]  GraphicShininess=75  GraphicOpacity=smiData.Solid(6).opacity  GeometryShape=FromFile  RectangleSize=[1 1]  RectangleSizeUnits=m  BrickDimensions=[1 1 1]  BrickDimensionUnits=m  CylinderRadius=1  CylinderRadiusUnits=m  CylinderLength=1  CylinderLengthUnits=m  SphereRadius=1  SphereRadiusUnits=m  EllipsoidRadii=[1 1 1]  EllipsoidRadiiUnits=m  ExtrusionCrossSection=[1 1; -1 1; -1 -1; 1 -1]  ExtrusionCrossSectionUnits=m  ExtrusionLength=1  ExtrusionLengthUnits=m  PolygonNumSides=3  PolygonOuterRadius=1  PolygonOuterRadiusUnits=m  ExtGeomFileType=STEP  ExtGeomFileName=Link6_默认_sldprt.STEP  ExtGeomFileUnits=m  RevolutionCrossSection=[1 1; 1 -1; 2 -1; 2 1]  RevolutionCrossSectionUnits=m  RevolutionExtent=Full  RevolutionAngle=180  RevolutionAngleUnits=deg
  Transform : sm_lib/Frames and Transforms/Rigid Transform  TranslationMethod=Cartesian  TranslationStandardOffset=0  TranslationLengthUnit=mm  TranslationStandardAxis=+Z  TranslationCartesianOffset=smiData.RigidTransform(12).translation  TranslationROffset=0  TranslationROffsetUnits=m  TranslationZOffset=0  TranslationZOffsetUnits=m  TranslationThetaOffset=0  TranslationThetaOffsetUnits=deg  RotationMethod=ArbitraryAxis  RotationAngleUnits=rad  RotationStandardAxis=+Z  RotationAngle=smiData.RigidTransform(12).angle  RotationArbitraryAxis=smiData.RigidTransform(12).axis  FollAlignAxisA=+X  BaseAlignAxisA=+Y  FollAlignAxisB=+Y  BaseAlignAxisB=+Z  RotationSequenceAxes=FollowerAxes  RotationSequence=XYX  RotationSequenceAngles=[0 0 0]  RotationSequenceAnglesUnits=deg  RotationMatrix=[1 0 0; 0 1 0; 0 0 1]
  F : PMIOPort  Side=Left
  connections:
  Solid/RConn1 -- ReferenceFrame/RConn1 -- Transform/LConn1
  Transform/RConn1 -- F/RConn1

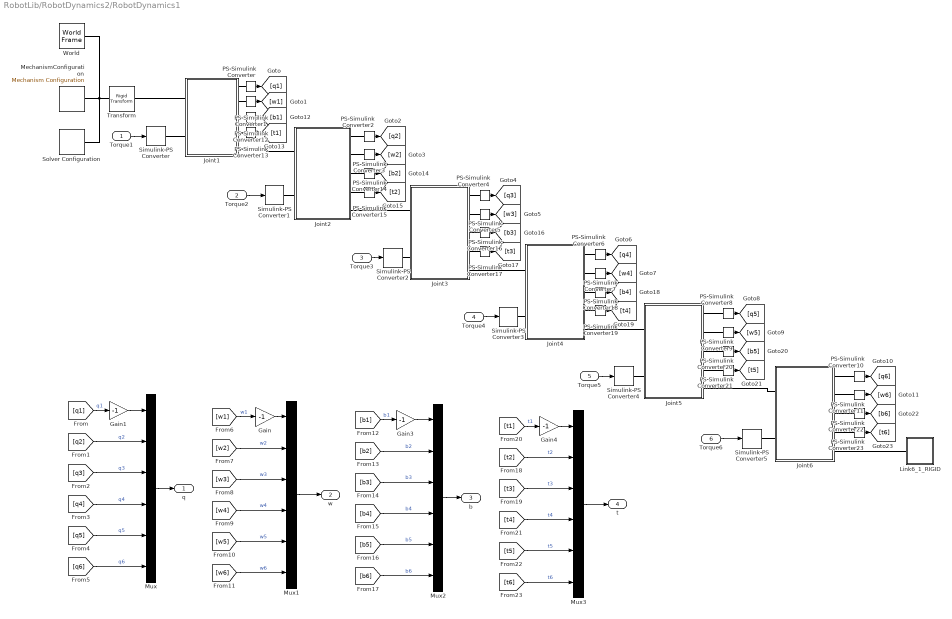
== system RobotLib/RobotDynamics2/RobotDynamics1 ==
  Torque1 : Inport
  Torque2 : Inport  Port=2
  Torque3 : Inport  Port=3
  Torque4 : Inport  Port=4
  Torque5 : Inport  Port=5
  Torque6 : Inport  Port=6
  Gain{,1,3..4} (4 alike) : Gain  Gain=-1
  Joint1 : Subsystem
  Joint2 : Subsystem
  Joint3 : Subsystem
  Joint4 : Subsystem
  Joint5 : Subsystem
  Joint6 : Subsystem
  Link6_1_RIGID : Subsystem
  MechanismConfiguration : sm_lib/Utilities/Mechanism Configuration  UniformGravity=Constant  GravityVector=[0 -9.80665 0]  GravityUnits=m/s^2  LinearizationDelta=0.001
  Mux{,1..3} (4 alike) : Mux  Inputs=6
  PS-Simulink Converter{,2,4,6,8,10} (6 alike) : nesl_utility/PS-Simulink Converter  PhysicalDomain=network_engine_domain  SubClassName=ps_output  LeftPortType=input  RightPortType=output  PseudoPeriodic=off  Frequencies=[]  Unit=deg  AffineConversion=off
  PS-Simulink Converter{1,3,5,7,9,11} (6 alike) : nesl_utility/PS-Simulink Converter  PhysicalDomain=network_engine_domain  SubClassName=ps_output  LeftPortType=input  RightPortType=output  PseudoPeriodic=off  Frequencies=[]  Unit=deg/s  AffineConversion=off
  PS-Simulink Converter{12,14,16,18,20,22} (6 alike) : nesl_utility/PS-Simulink Converter  PhysicalDomain=network_engine_domain  SubClassName=ps_output  LeftPortType=input  RightPortType=output  PseudoPeriodic=off  Frequencies=[]  Unit=deg/s^2  AffineConversion=off
  PS-Simulink Converter{13,15,17,19,21,23} (6 alike) : nesl_utility/PS-Simulink Converter  PhysicalDomain=network_engine_domain  SubClassName=ps_output  LeftPortType=input  RightPortType=output  PseudoPeriodic=off  Frequencies=[]  Unit=N*m  AffineConversion=off
  Simulink-PS Converter{,1..5} (6 alike) : nesl_utility/Simulink-PS Converter  PhysicalDomain=network_engine_domain  SubClassName=ps_input  LeftPortType=input  RightPortType=output  PseudoPeriodic=off  Frequencies=[]  NoiseDistribution=none  NoiseParameters=[]  Unit=N*m  AffineConversion=off  FilteringAndDerivatives=provide  SimscapeFilterOrder=2  InputFilterTimeConstant=0.001  UdotUserProvided=0
  Solver Configuration : nesl_utility/Solver Configuration  PhysicalDomain=network_engine_domain  SubClassName=solver  LeftPortType=input  RightPortType=generic  Tones=[]  Harmonics=[]  SimulateNoise=off  Profile=off  UseLocalSampling=off  EnableSwitchedLinearOptims=on  FrequencyDomain=off  UseCCode=off  RelTol=0.001  AbsTol=1e-06  MinStep=1e-09  ToWorkspace=off  RevertToSquareIcSolve=off  NumHomotopyIterations=100  PhasorMode=off  PhasorModeNumHarmonics=1  DoDC=off  ResidualTolerance=1e-09  UseLocalSolver=off  LocalSolverChoice=NE_BACKWARD_EULER_ADVANCER  LocalSolverSampleTime=0.001  DoFixedCost=off  MaxNonlinIter=3  MaxModeIter=2  LinearAlgebra=auto  EquationFormulation=NE_TIME_EF  DelaysMemoryBudget=1024  AutomaticFiltering=on  FilteringTimeConstant=0.001  PartitionStorageMethod=AS_NEEDED  PartitionMemoryBudget=1024
  Transform : sm_lib/Frames and Transforms/Rigid Transform  TranslationMethod=Cartesian  TranslationStandardOffset=0  TranslationLengthUnit=mm  TranslationStandardAxis=+Z  TranslationCartesianOffset=smiData.RigidTransform(14).translation  TranslationROffset=0  TranslationROffsetUnits=m  TranslationZOffset=0  TranslationZOffsetUnits=m  TranslationThetaOffset=0  TranslationThetaOffsetUnits=deg  RotationMethod=ArbitraryAxis  RotationAngleUnits=rad  RotationStandardAxis=+Z  RotationAngle=smiData.RigidTransform(14).angle  RotationArbitraryAxis=smiData.RigidTransform(14).axis  FollAlignAxisA=+X  BaseAlignAxisA=+Y  FollAlignAxisB=+Y  BaseAlignAxisB=+Z  RotationSequenceAxes=FollowerAxes  RotationSequence=XYX  RotationSequenceAngles=[0 0 0]  RotationSequenceAnglesUnits=deg  RotationMatrix=[1 0 0; 0 1 0; 0 0 1]
  World : sm_lib/Frames and Transforms/World Frame
  q : Outport  VectorParamsAs1DForOutWhenUnconnected=on
  w : Outport  Port=2  VectorParamsAs1DForOutWhenUnconnected=on
  b : Outport  Port=3  VectorParamsAs1DForOutWhenUnconnected=on
  t : Outport  Port=4  VectorParamsAs1DForOutWhenUnconnected=on
  wires:
  Gain4/1 -> Mux3/1
  Torque1/1 -> Simulink-PS Converter/1
  [t6] -> Mux3/6  "t6"
  [t5] -> Mux3/5  "t5"
  [t4] -> Mux3/4  "t4"
  [t3] -> Mux3/3  "t3"
  [t2] -> Mux3/2  "t2"
  [b6] -> Mux2/6  "b6"
  [b5] -> Mux2/5  "b5"
  [b4] -> Mux2/4  "b4"
  [b3] -> Mux2/3  "b3"
  [b2] -> Mux2/2  "b2"
  Mux2/1 -> b/1
  [t1] -> Gain4/1  "t1"
  Mux3/1 -> t/1
  [b1] -> Gain3/1  "b1"
  Gain3/1 -> Mux2/1
  PS-Simulink Converter22/1 -> [b6]
  PS-Simulink Converter23/1 -> [t6]
  PS-Simulink Converter21/1 -> [t5]
  PS-Simulink Converter20/1 -> [b5]
  PS-Simulink Converter18/1 -> [b4]
  PS-Simulink Converter19/1 -> [t4]
  PS-Simulink Converter17/1 -> [t3]
  PS-Simulink Converter16/1 -> [b3]
  PS-Simulink Converter14/1 -> [b2]
  PS-Simulink Converter15/1 -> [t2]
  PS-Simulink Converter13/1 -> [t1]
  PS-Simulink Converter12/1 -> [b1]
  Gain1/1 -> Mux/1
  Gain/1 -> Mux1/1
  Torque6/1 -> Simulink-PS Converter5/1
  Torque5/1 -> Simulink-PS Converter4/1
  Torque4/1 -> Simulink-PS Converter3/1
  Torque3/1 -> Simulink-PS Converter2/1
  Torque2/1 -> Simulink-PS Converter1/1
  PS-Simulink Converter3/1 -> [w2]
  [w3] -> Mux1/3  "w3"
  [q1] -> Gain1/1  "q1"
  [q3] -> Mux/3  "q3"
  PS-Simulink Converter2/1 -> [q2]
  Mux1/1 -> w/1
  PS-Simulink Converter8/1 -> [q5]
  PS-Simulink Converter11/1 -> [w6]
  [q4] -> Mux/4  "q4"
  PS-Simulink Converter7/1 -> [w4]
  [w6] -> Mux1/6  "w6"
  PS-Simulink Converter10/1 -> [q6]
  [q2] -> Mux/2  "q2"
  PS-Simulink Converter1/1 -> [w1]
  [w2] -> Mux1/2  "w2"
  PS-Simulink Converter9/1 -> [w5]
  PS-Simulink Converter5/1 -> [w3]
  PS-Simulink Converter4/1 -> [q3]
  [w5] -> Mux1/5  "w5"
  [w1] -> Gain/1  "w1"
  [q6] -> Mux/6  "q6"
  PS-Simulink Converter/1 -> [q1]
  [w4] -> Mux1/4  "w4"
  PS-Simulink Converter6/1 -> [q4]
  Mux/1 -> q/1
  [q5] -> Mux/5  "q5"
  connections:
  Joint1/LConn2 -- Simulink-PS Converter/RConn1
  Joint6/RConn3 -- PS-Simulink Converter22/LConn1
  PS-Simulink Converter23/LConn1 -- Joint6/RConn4
  PS-Simulink Converter21/LConn1 -- Joint5/RConn4
  PS-Simulink Converter20/LConn1 -- Joint5/RConn3
  PS-Simulink Converter19/LConn1 -- Joint4/RConn4
  PS-Simulink Converter18/LConn1 -- Joint4/RConn3
  Joint3/RConn4 -- PS-Simulink Converter17/LConn1
  PS-Simulink Converter16/LConn1 -- Joint3/RConn3
  PS-Simulink Converter14/LConn1 -- Joint2/RConn3
  PS-Simulink Converter15/LConn1 -- Joint2/RConn4
  PS-Simulink Converter13/LConn1 -- Joint1/RConn4
  PS-Simulink Converter12/LConn1 -- Joint1/RConn3
  Simulink-PS Converter2/RConn1 -- Joint3/LConn2
  Joint2/LConn1 -- Joint1/RConn5
  Joint5/LConn2 -- Simulink-PS Converter4/RConn1
  PS-Simulink Converter2/LConn1 -- Joint2/RConn1
  Simulink-PS Converter1/RConn1 -- Joint2/LConn2
  Simulink-PS Converter5/RConn1 -- Joint6/LConn2
  Link6_1_RIGID/LConn1 -- Joint6/RConn5
  Joint5/LConn1 -- Joint4/RConn5
  Joint3/LConn1 -- Joint2/RConn5
  Joint6/LConn1 -- Joint5/RConn5
  Joint1/RConn1 -- PS-Simulink Converter/LConn1
  PS-Simulink Converter4/LConn1 -- Joint3/RConn1
  Simulink-PS Converter3/RConn1 -- Joint4/LConn2
  PS-Simulink Converter8/LConn1 -- Joint5/RConn1
  Joint1/LConn1 -- Transform/RConn1
  PS-Simulink Converter3/LConn1 -- Joint2/RConn2
  Joint1/RConn2 -- PS-Simulink Converter1/LConn1
  Joint3/RConn5 -- Joint4/LConn1
  World/RConn1 -- Solver Configuration/RConn1 -- MechanismConfiguration/RConn1 -- Transform/LConn1
  PS-Simulink Converter5/LConn1 -- Joint3/RConn2
  PS-Simulink Converter9/LConn1 -- Joint5/RConn2
  Joint4/RConn1 -- PS-Simulink Converter6/LConn1
  Joint4/RConn2 -- PS-Simulink Converter7/LConn1
  PS-Simulink Converter11/LConn1 -- Joint6/RConn2
  Joint6/RConn1 -- PS-Simulink Converter10/LConn1

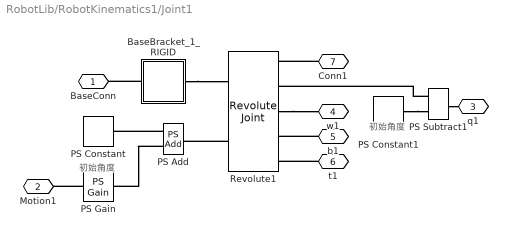
== system RobotLib/RobotKinematics1/Joint1 ==
  note: 初始角度
  note: 初始角度
  BaseBracket_1_RIGID : Subsystem
  PS Add : fl_lib/Physical Signals/Functions/PS Add
  PS Constant : fl_lib/Physical Signals/Sources/PS Constant  constant=-pi/2
  PS Constant1 : fl_lib/Physical Signals/Sources/PS Constant  constant=-pi/2
  PS Gain : fl_lib/Physical Signals/Functions/PS Gain  gain=-1
  PS Subtract1 : fl_lib/Physical Signals/Functions/PS Subtract
      settings: SourceProductName=Simscape
  Revolute1 : sm_lib/Joints/Revolute Joint  SenseConstraintForce=off  SenseConstraintForceX=off  SenseConstraintForceY=off  SenseConstraintForceZ=off  SenseConstraintTorque=off  SenseConstraintTorqueX=off  SenseConstraintTorqueY=off  SenseConstraintTorqueZ=off  SenseTotalForce=off  SenseTotalForceX=off  SenseTotalForceY=off  SenseTotalForceZ=off  SenseTotalTorque=off  SenseTotalTorqueX=off  SenseTotalTorqueY=off  SenseTotalTorqueZ=off  CompositeWrenchDir=FollowerOnBase  CompositeWrenchFrame=BaseFrame  EquilibriumPosition=0  EquilibriumPositionUnits=rad  SpringStiffness=0  SpringStiffnessUnits=N*m/rad  DampingCoefficient=0  DampingCoefficientUnits=N*m/(rad/s)  TorqueActuationMode=ComputedTorque  MotionActuationMode=InputMotion  SensePosition=on  SenseVelocity=on  SenseAcceleration=on  SenseTorqueForce=on  PositionTargetSpecify=on  PositionTargetPriority=Low  PositionTargetValue=smiData.RevoluteJoint(2).Rz.Pos  PositionTargetValueUnits=deg  VelocityTargetSpecify=off  VelocityTargetPriority=High  VelocityTargetValue=0  VelocityTargetValueUnits=deg/s
  BaseConn : PMIOPort  Side=Left
  Motion1 : PMIOPort  Port=2  Side=Left
  q1 : PMIOPort  Port=3  Side=Right
  w1 : PMIOPort  Port=4  Side=Right
  b1 : PMIOPort  Port=5  Side=Right
  t1 : PMIOPort  Port=6  Side=Right
  Conn1 : PMIOPort  Port=7  Side=Right
  connections:
  t1/RConn1 -- Revolute1/RConn5
  b1/RConn1 -- Revolute1/RConn4
  Revolute1/RConn3 -- w1/RConn1
  PS Subtract1/RConn1 -- q1/RConn1
  PS Constant1/RConn1 -- PS Subtract1/LConn2
  PS Subtract1/LConn1 -- Revolute1/RConn2
  BaseBracket_1_RIGID/LConn1 -- BaseConn/RConn1
  Conn1/RConn1 -- Revolute1/RConn1
  BaseBracket_1_RIGID/RConn1 -- Revolute1/LConn1
  Revolute1/LConn2 -- PS Add/RConn1
  PS Add/LConn1 -- PS Constant/RConn1
  PS Gain/LConn1 -- Motion1/RConn1
  PS Add/LConn2 -- PS Gain/RConn1

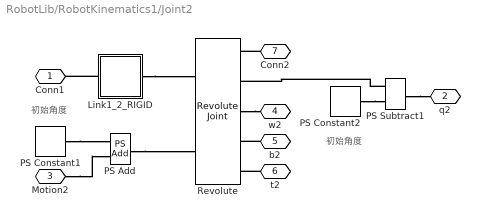
== system RobotLib/RobotKinematics1/Joint2 ==
  note: 初始角度
  note: 初始角度
  Link1_2_RIGID : Subsystem
  PS Add : fl_lib/Physical Signals/Functions/PS Add
  PS Constant1 : fl_lib/Physical Signals/Sources/PS Constant  constant=-pi/2
  PS Constant2 : fl_lib/Physical Signals/Sources/PS Constant  constant=-pi/2
  PS Subtract1 : fl_lib/Physical Signals/Functions/PS Subtract
      settings: SourceProductName=Simscape
  Revolute : sm_lib/Joints/Revolute Joint  SenseConstraintForce=off  SenseConstraintForceX=off  SenseConstraintForceY=off  SenseConstraintForceZ=off  SenseConstraintTorque=off  SenseConstraintTorqueX=off  SenseConstraintTorqueY=off  SenseConstraintTorqueZ=off  SenseTotalForce=off  SenseTotalForceX=off  SenseTotalForceY=off  SenseTotalForceZ=off  SenseTotalTorque=off  SenseTotalTorqueX=off  SenseTotalTorqueY=off  SenseTotalTorqueZ=off  CompositeWrenchDir=FollowerOnBase  CompositeWrenchFrame=BaseFrame  EquilibriumPosition=0  EquilibriumPositionUnits=rad  SpringStiffness=0  SpringStiffnessUnits=N*m/rad  DampingCoefficient=0  DampingCoefficientUnits=N*m/(rad/s)  TorqueActuationMode=ComputedTorque  MotionActuationMode=InputMotion  SensePosition=on  SenseVelocity=on  SenseAcceleration=on  SenseTorqueForce=on  PositionTargetSpecify=on  PositionTargetPriority=Low  PositionTargetValue=smiData.RevoluteJoint(1).Rz.Pos  PositionTargetValueUnits=deg  VelocityTargetSpecify=off  VelocityTargetPriority=High  VelocityTargetValue=0  VelocityTargetValueUnits=deg/s
  Conn1 : PMIOPort  Side=Left
  q2 : PMIOPort  Port=2  Side=Right
  Motion2 : PMIOPort  Port=3  Side=Left
  w2 : PMIOPort  Port=4  Side=Right
  b2 : PMIOPort  Port=5  Side=Right
  t2 : PMIOPort  Port=6  Side=Right
  Conn2 : PMIOPort  Port=7  Side=Right
  connections:
  t2/RConn1 -- Revolute/RConn5
  b2/RConn1 -- Revolute/RConn4
  PS Subtract1/RConn1 -- q2/RConn1
  PS Constant2/RConn1 -- PS Subtract1/LConn2
  Revolute/RConn3 -- w2/RConn1
  PS Subtract1/LConn1 -- Revolute/RConn2
  Conn2/RConn1 -- Revolute/RConn1
  Link1_2_RIGID/RConn1 -- Revolute/LConn1
  Link1_2_RIGID/LConn1 -- Conn1/RConn1
  PS Constant1/RConn1 -- PS Add/LConn1
  Motion2/RConn1 -- PS Add/LConn2
  PS Add/RConn1 -- Revolute/LConn2
